simulink model "DopplerDynamics_Ethernet_PDR"  (R2023b)
settings: Solver=VariableStepDiscrete  StartTime=0.0  StopTime=SIM_TIME_S  RelTol=1e-3
values from neighbouring files (symbols this model uses):
  DOPPLER_PACKET_PERIOD_S = AVERAGE_PAYLOAD_BYTES * 8 / DOPPLER_APP_RATE_BPS    [dd_network_init.m]
  IVUS_PACKET_PERIOD_S = AVERAGE_PAYLOAD_BYTES * 8 / IVUS_APP_RATE_BPS    [dd_network_init.m]
undefined symbols (not defined in the file or in its folder): m, n
settings Model: Creator=micae  LastModifiedBy=micae

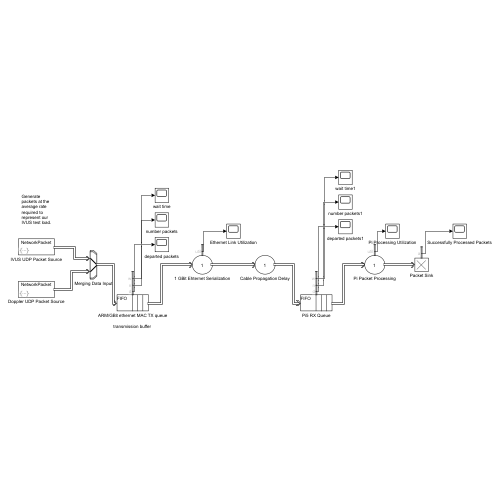
[thumbnail: Simulink's stored preview of the top-level diagram]
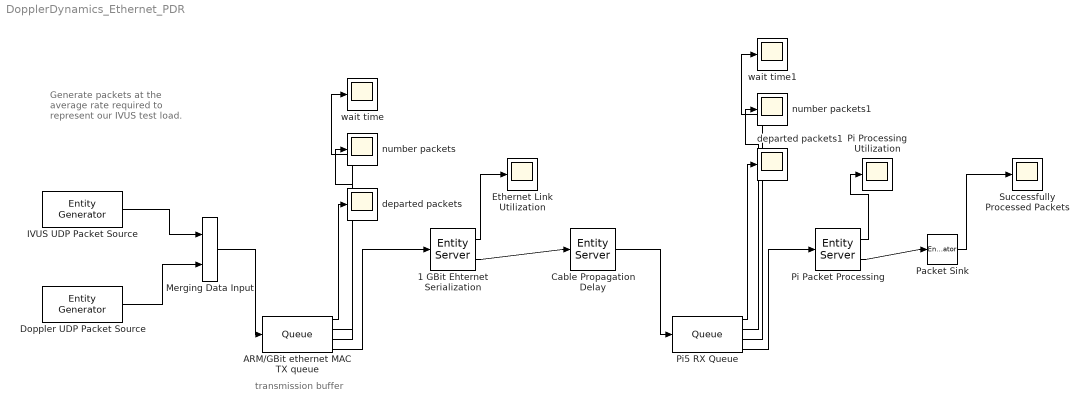
== system DopplerDynamics_Ethernet_PDR ==
  note: transmission buffer
  note: Generate packets at the average rate required to represent our IVUS test load.
  1 GBit Ehternet Serialization : EntityServer  InputPortMessageModes=m  OutputPortMessageModes=n,m  Capacity=1  ServiceTimeSource=Attribute  ServiceTimeAttributeName=TxTime  Utilization=on
      settings: OutputPortMap=o5,o9
  ARM/GBit ethernet MAC TX queue : Queue  InputPortMessageModes=m  OutputPortMessageModes=n,n,n,m  Capacity=TX_QUEUE_CAPACITY  NumberEntitiesDeparted=on  NumberEntitiesInBlock=on  AverageWait=on
      settings: OutputPortMap=o0,o1,o2,o5
  Cable Propagation Delay : EntityServer  InputPortMessageModes=m  OutputPortMessageModes=m  Capacity=1  ServiceTimeValue=PROPAGATION_DELAY_S
  Doppler UDP Packet Source : EntityGenerator  OutputPortMessageModes=m  Period=DOPPLER_PACKET_PERIOD_S  GenerateAction=|  AttributeName=StreamType|Sequence|FrameID|PacketIndex|PacketsInFrame|PayloadBytes|WireBytes|TxTime|Route  AttributeInitialValue=1|0|0|0|12|1400|1498|FULL_TX_TIME_S|1  EntityType=Structured  EntityTypeName=NetworkPacket
      | persistent dopplerSeq
      | 
      | if isempty(dopplerSeq)
      |     dopplerSeq = 0;
      | end
      | 
      | entity.StreamType = 2;
      | 
      | entity.Sequence = dopplerSeq;
      | 
      | entity.FrameID = ...
      |     floor(dopplerSeq / PACKETS_PER_DMA_BLOCK);
      | 
      | entity.PacketIndex = ...
      |     mod(dopplerSeq, PACKETS_PER_DMA_BLOCK);
      | 
      | entity.PacketsInFrame = ...
      |     PACKETS_PER_DMA_BLOCK;
      | 
      | if entity.PacketIndex == ...
      |         PACKETS_PER_DMA_BLOCK - 1
      | 
      |     entity.PayloadBytes = ...
      |         LAST_PAYLOAD_BYTES;
      | 
      | else
      | 
      |     entity.PayloadBytes = ...
      |         SENSOR_PAYLOAD_BYTES;
      | 
      | end
      | 
      | entity.WireBytes = ...
      |     entity.PayloadBytes + ...
      |     OVERHEAD_BYTE_TIMES;
      | 
      | entity.TxTime = ...
      |     entity.WireBytes * 8 / ...
      |     LINK_RATE_BPS;
      | 
      | entity.Route = 1;
      | 
      | dopplerSeq = dopplerSeq + 1;
  Ethernet Link Utilization : Scope
  IVUS UDP Packet Source : EntityGenerator  OutputPortMessageModes=m  Period=IVUS_PACKET_PERIOD_S  GenerateAction=|  AttributeName=StreamType|Sequence|FrameID|PacketIndex|PacketsInFrame|PayloadBytes|WireBytes|TxTime|Route  AttributeInitialValue=1|0|0|0|12|1400|1498|FULL_TX_TIME_S|1  EntityType=Structured  EntityTypeName=NetworkPacket
      | persistent seq
      | 
      | if isempty(seq)
      |     seq = 0;
      | end
      | 
      | entity.StreamType = 1;
      | 
      | entity.Sequence = seq;
      | 
      | entity.FrameID = ...
      |     floor(seq / PACKETS_PER_DMA_BLOCK);
      | 
      | entity.PacketIndex = ...
      |     mod(seq, PACKETS_PER_DMA_BLOCK);
      | 
      | entity.PacketsInFrame = ...
      |     PACKETS_PER_DMA_BLOCK;
      | 
      | if entity.PacketIndex == ...
      |         PACKETS_PER_DMA_BLOCK - 1
      | 
      |     entity.PayloadBytes = ...
      |         LAST_PAYLOAD_BYTES;
      | 
      | else
      | 
      |     entity.PayloadBytes = ...
      |         SENSOR_PAYLOAD_BYTES;
      | 
      | end
      | 
      | entity.WireBytes = ...
      |     entity.PayloadBytes + ...
      |     OVERHEAD_BYTE_TIMES;
      | 
      | entity.TxTime = ...
      |     entity.WireBytes * 8 / ...
      |     LINK_RATE_BPS;
      | 
      | entity.Route = 1;
      | 
      | seq = seq + 1;
  Merging Data Input : EntityInputSwitch  InputPortMessageModes=m,m  OutputPortMessageModes=m
  Packet Sink : EntityTerminator  InputPortMessageModes=m  NumberEntitiesArrived=on
      settings: OutputPortMap=o0
  Pi Packet Processing : EntityServer  InputPortMessageModes=m  OutputPortMessageModes=n,m  Capacity=1  ServiceTimeValue=PI_PROCESS_TIME_S  Utilization=on
      settings: OutputPortMap=o5,o9
  Pi Processing Utilization : Scope
  Pi5 RX Queue : Queue  InputPortMessageModes=m  OutputPortMessageModes=n,n,n,m  Capacity=RX_QUEUE_CAPACITY  NumberEntitiesDeparted=on  NumberEntitiesInBlock=on  AverageWait=on
      settings: OutputPortMap=o0,o1,o2,o5
  Successfully Processed Packets : Scope
  departed packets : Scope
  departed packets1 : Scope
  number packets : Scope
  number packets1 : Scope
  wait time : Scope
  wait time1 : Scope
  wires:
  IVUS UDP Packet Source/1 -> Merging Data Input/1
  Doppler UDP Packet Source/1 -> Merging Data Input/2
  Merging Data Input/1 -> ARM/GBit ethernet MAC TX queue/1
  ARM/GBit ethernet MAC TX queue/4 -> 1 GBit Ehternet Serialization/1
  1 GBit Ehternet Serialization/2 -> Cable Propagation Delay/1
  Cable Propagation Delay/1 -> Pi5 RX Queue/1
  Pi5 RX Queue/4 -> Pi Packet Processing/1
  Pi Packet Processing/2 -> Packet Sink/1
  1 GBit Ehternet Serialization/1 -> Ethernet Link Utilization/1
  Pi Packet Processing/1 -> Pi Processing Utilization/1
  Packet Sink/1 -> Successfully Processed Packets/1
  ARM/GBit ethernet MAC TX queue/1 -> departed packets/1
  ARM/GBit ethernet MAC TX queue/2 -> number packets/1
  ARM/GBit ethernet MAC TX queue/3 -> wait time/1
  Pi5 RX Queue/1 -> departed packets1/1
  Pi5 RX Queue/2 -> number packets1/1
  Pi5 RX Queue/3 -> wait time1/1
